simulink library "two_norm"  (R2018b)
settings: Solver=VariableStepAuto  StartTime=0.0  StopTime=10.0  RelTol=1e-3
settings Model: Creator=colem  LastModifiedBy=colem

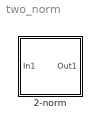
== system two_norm ==
  2-norm : Subsystem

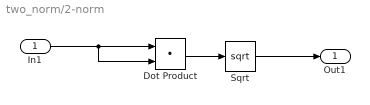
== system two_norm/2-norm ==
  In1 : Inport
  Dot Product : DotProduct  InputSameDT=on  OutDataTypeStr=Inherit: Inherit via internal rule
  Sqrt : Sqrt  SaturateOnIntegerOverflow=on
  Out1 : Outport
  wires:
  In1/1 -> Dot Product/2, Dot Product/1
  Sqrt/1 -> Out1/1
  Dot Product/1 -> Sqrt/1
